simulink model "mpc_varbounds"  (Simulink 6.6)
settings: Solver=ode3  StartTime=0.0  StopTime=Tsim  RelTol=1e-3
values from neighbouring files (symbols this model uses):
  Tsim = 20    [mpcvarbounds.m]
libraries: simulink x3, cstblocks x1, mpclib x1
settings Model: Creator=Alberto Bemporad  LastModifiedBy=rchen  ExtModeTrigMode=oneshot  ExtModeArmWhenConnect=off
settings DataIOCC: LimitDataPoints=off  SignalLoggingName=sigsOut
settings OptimizationCC: BooleanDataType=off
settings DebuggingCC: SignalResolutionControl=TryResolveAllWithWarning  SolverPrmCheckMsg=none  MultiTaskDSMMsg=warning  MultiTaskCondExecSysMsg=none  StrictBusMsg=None
settings HardwareCC: TargetEndianess=LittleEndian  TargetHWDeviceType=MATLAB Host  ProdEqTarget=off
settings RTWCC: IncludeERTFirstTime=on

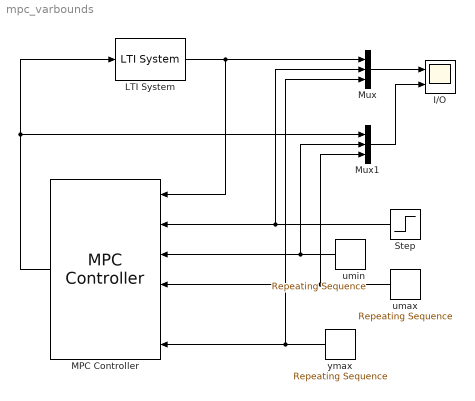
== system mpc_varbounds ==
  I/O : Scope  NumInputPorts=2
      settings: TimeRange=20  YMin=0~1.5  YMax=1.5~4
  LTI System : cstblocks/LTI System  SystemSampleTime=-1  sys=plant  IC=[]
  MPC Controller : mpclib/MPC Controller  Orientation=left  SystemSampleTime=-1  mpcobj=mpc1  n_mv=0  x0=[]  ref_from_ws=off  ref_signal_name=[]  ref_preview=on  md_from_ws=off  md_signal_name=[]  md_preview=on  from_project=off  md_inport=off  mv_inport=off  lims_inport=on  project_file=MPCtask.mat
  Mux : Mux  Inputs=3
  Mux1 : Mux  Inputs=3
  Step : Step  Orientation=left  Time=0  Before=1  SampleTime=0
  umax : simulink/Sources/Repeating Sequence  Orientation=left  SystemSampleTime=-1  rep_seq_t=[0 1 6 Tsim]  rep_seq_y=[3 2 3 3]
  umin : simulink/Sources/Repeating Sequence  Orientation=left  SystemSampleTime=-1  rep_seq_t=[0 2 4 Tsim]  rep_seq_y=[1.5 2 2.5 2.5]
  ymax : simulink/Sources/Repeating Sequence  Orientation=left  SystemSampleTime=-1  rep_seq_t=[0 1 10 15 Tsim]  rep_seq_y=[1.2 1.2 0.9 1.2 1]
  wires:
  Mux/1 -> I/O/1
  MPC Controller/1 -> LTI System/1, Mux1/1
  Step/1 -> Mux/2, MPC Controller/2
  Mux1/1 -> I/O/2
  umin/1 -> Mux1/2, MPC Controller/3
  umax/1 -> Mux1/3, MPC Controller/4
  LTI System/1 -> Mux/1, MPC Controller/1
  ymax/1 -> MPC Controller/6, Mux/3
